simulink model "SWC_FDC_type"  (R2021b)
settings: Solver=FixedStepDiscrete  StartTime=0.0  StopTime=10.0  FixedStep=0.001  RelTol=1e-3
values from neighbouring files (symbols this model uses):
  DID_VCUKey = uint16(0x0202)    [vcu_local_hdr.m]
  DID_XWD = uint16(513)    [vcu_local_hdr.m]
  DIDLen_APSFunConfig = uint16(16)    [vcu_local_hdr.m]
  DIDLen_AutoLock = uint16(1)    [vcu_local_hdr.m]
  DIDLen_DKCKey = uint16(8)    [vcu_local_hdr.m]
  DIDLen_DRLDis = uint16(1)    [vcu_local_hdr.m]
  DIDLen_DynoMode = uint16(1)    [vcu_local_hdr.m]
  DIDLen_FMHTimer = uint16(1)    [vcu_local_hdr.m]
  DIDLen_LFLowPresThre = uint16(1)    [vcu_local_hdr.m]
  DIDLen_LFSensorID = uint16(4)    [vcu_local_hdr.m]
  DIDLen_LRLowPresThre = uint16(1)    [vcu_local_hdr.m]
  DIDLen_LRSensorID = uint16(4)    [vcu_local_hdr.m]
  DIDLen_RFLowPresThre = uint16(1)    [vcu_local_hdr.m]
  DIDLen_RFSensorID = uint16(4)    [vcu_local_hdr.m]
  DIDLen_RRLowPresThre = uint16(1)    [vcu_local_hdr.m]
  DIDLen_RRSensorID = uint16(4)    [vcu_local_hdr.m]
  DIDLen_SensorMode = uint16(1)    [vcu_local_hdr.m]
  DIDLen_TireSize = uint16(16)    [vcu_local_hdr.m]
  DIDLen_TPMSLearnSta = uint16(1)    [vcu_local_hdr.m]
  DIDLen_TurnLampFLThreCurr = uint16(1)    [vcu_local_hdr.m]
  DIDLen_TurnLampFRThreCurr = uint16(1)    [vcu_local_hdr.m]
  DIDLen_TurnLampRLThreCurr = uint16(1)    [vcu_local_hdr.m]
  DIDLen_TurnLampRRThreCurr = uint16(1)    [vcu_local_hdr.m]
  DIDLen_USSConfig = uint16(16)    [vcu_local_hdr.m]
  DIDLen_WhlPres = uint16(4)    [vcu_local_hdr.m]
  DIDLen_WhlSensorBattSta = uint16(1)    [vcu_local_hdr.m]
  DIDLen_WhlTmp = uint16(4)    [vcu_local_hdr.m]
  DIDLen_XWDMode = uint16(1)    [vcu_local_hdr.m]
  DIDNum_APSFunConfig = uint16(0x0903)    [vcu_local_hdr.m]
  DIDNum_AutoLock = uint16(0x0306)    [vcu_local_hdr.m]
  DIDNum_DKCKey = uint16(0x0202)    [vcu_local_hdr.m]
  DIDNum_DRLDis = uint16(0x0307)    [vcu_local_hdr.m]
  DIDNum_DynoMode = uint16(0x0203)    [vcu_local_hdr.m]
  DIDNum_FMHTimer = uint16(0x0305)    [vcu_local_hdr.m]
  DIDNum_LFLowPresThre = uint16(0x0B08)    [vcu_local_hdr.m]
  DIDNum_LFSensorID = uint16(0x0B01)    [vcu_local_hdr.m]
  DIDNum_LRLowPresThre = uint16(0x0B0A)    [vcu_local_hdr.m]
  DIDNum_LRSensorID = uint16(0x0B03)    [vcu_local_hdr.m]
  DIDNum_RFLowPresThre = uint16(0x0B09)    [vcu_local_hdr.m]
  DIDNum_RFSensorID = uint16(0x0B02)    [vcu_local_hdr.m]
  DIDNum_RRLowPresThre = uint16(0x0B0B)    [vcu_local_hdr.m]
  DIDNum_RRSensorID = uint16(0x0B04)    [vcu_local_hdr.m]
  DIDNum_SensorMode = uint16(0x0B0C)    [vcu_local_hdr.m]
  DIDNum_TireSize = uint16(0x0902)    [vcu_local_hdr.m]
  DIDNum_TPMSLearnSta = uint16(0x0B0D)    [vcu_local_hdr.m]
  DIDNum_TurnLampFLThreCurr = uint16(0x0303)    [vcu_local_hdr.m]
  DIDNum_TurnLampFRThreCurr = uint16(0x0301)    [vcu_local_hdr.m]
  DIDNum_TurnLampRLThreCurr = uint16(0x0304)    [vcu_local_hdr.m]
  DIDNum_TurnLampRRThreCurr = uint16(0x0302)    [vcu_local_hdr.m]
  DIDNum_USSConfig = uint16(0x0901)    [vcu_local_hdr.m]
  DIDNum_WhlPres = uint16(0x0B05)    [vcu_local_hdr.m]
  DIDNum_WhlSensorBattSta = uint16(0x0B07)    [vcu_local_hdr.m]
  DIDNum_WhlTmp = uint16(0x0B06)    [vcu_local_hdr.m]
  DIDNum_XWDMode = uint16(0x0201)    [vcu_local_hdr.m]
  DIDVCUKeyLength = uint16(8)    [vcu_local_hdr.m]
  ENUM_DRIVETRAIN_AWD = uint8(  2  )    [vcu_local_hdr.m]
  ENUM_DRIVETRAIN_FWD = uint8(  1  )    [vcu_local_hdr.m]
  ENUM_DRIVETRAIN_RWD = uint8(  0  )    [vcu_local_hdr.m]
  ENUM_REGENLEVEL_INVALID = uint8(  7  )    [vcu_local_hdr.m]
  ENUM_REGENLEVEL_LV1 = uint8(  1  )    [vcu_local_hdr.m]
  ENUM_REGENLEVEL_LV2 = uint8(  2  )    [vcu_local_hdr.m]
  ENUM_REGENLEVEL_LV3 = uint8(  3  )    [vcu_local_hdr.m]
  ENUM_REGENLEVEL_LV4 = uint8(  4  )    [vcu_local_hdr.m]
  ENUM_REGENLEVEL_LV5 = uint8(  5  )    [vcu_local_hdr.m]
  ENUM_REGENLEVEL_OFF = uint8(  0  )    [vcu_local_hdr.m]
  ENUM_REGENLEVEL_OPD = uint8(  6  )    [vcu_local_hdr.m]
  ENUM_TPMSLearnStatus_LEARNED = uint8(  1  )    [vcu_local_hdr.m]
  ENUM_TPMSLearnStatus_LEARNFAIL = uint8(  2  )    [vcu_local_hdr.m]
  ENUM_TPMSLearnStatus_NOTLEARN = uint8(  0  )    [vcu_local_hdr.m]
  ENUM_TPMSSTA_FAT = uint8(  8  )    [vcu_local_hdr.m]
  ENUM_TPMSSTA_LOWBATTERY = uint8(  2  )    [vcu_local_hdr.m]
  FALSE = boolean( 0 )    [vcu_local_hdr.m]
  ONE_INT = uint8(1)    [vcu_local_hdr.m]
  P_boolean = 0.0    [APPTypes.sldd]
  TRUE = boolean( 1 )    [vcu_local_hdr.m]
  ZERO_FLOAT = single(0)    [vcu_local_hdr.m]
  ZERO_INT = uint8(0)    [vcu_local_hdr.m]
undefined symbols (not defined in the file or in its folder): f32_ApsOutVehSpdSig, KHAL_DKCDecryptEnable_flg_ovrdflg, KHAL_DKCDecryptEnable_flg_ovrdval, KHAL_RandomNumberY1_enum, KHAL_RandomNumberY2_enum, KHAL_RandomNumberY_ovrdflg, KHAL_THCMAPTCWarningDTC_flg_ovrdflg, KHAL_THCMAPTCWarningDTC_flg_ovrdval, KHAL_TPMSRESBUTT_flg_ovrdflg, KHAL_TPMSRESBUTT_flg_ovrdval, R_DIDWriteCDD_CSOP_DIDSet_APSFunConfig, R_DIDWriteCDD_CSOP_DIDSet_AutoLock, R_DIDWriteCDD_CSOP_DIDSet_DKCKey, R_DIDWriteCDD_CSOP_DIDSet_DRLDis, R_DIDWriteCDD_CSOP_DIDSet_DynoMode, R_DIDWriteCDD_CSOP_DIDSet_FMHTimer, R_DIDWriteCDD_CSOP_DIDSet_LFLowPresThre, R_DIDWriteCDD_CSOP_DIDSet_LFSensorID, R_DIDWriteCDD_CSOP_DIDSet_LRLowPresThre, R_DIDWriteCDD_CSOP_DIDSet_LRSensorID, R_DIDWriteCDD_CSOP_DIDSet_RFLowPresThre, R_DIDWriteCDD_CSOP_DIDSet_RFSensorID, R_DIDWriteCDD_CSOP_DIDSet_RRLowPresThre, R_DIDWriteCDD_CSOP_DIDSet_RRSensorID, R_DIDWriteCDD_CSOP_DIDSet_SensorMode, R_DIDWriteCDD_CSOP_DIDSet_TireSize, R_DIDWriteCDD_CSOP_DIDSet_TPMSLearnSta, R_DIDWriteCDD_CSOP_DIDSet_TurnLampFLThreCurr, R_DIDWriteCDD_CSOP_DIDSet_TurnLampFRThreCurr, R_DIDWriteCDD_CSOP_DIDSet_TurnLampRLThreCurr, R_DIDWriteCDD_CSOP_DIDSet_TurnLampRRThreCurr, R_DIDWriteCDD_CSOP_DIDSet_USSConfig, R_DIDWriteCDD_CSOP_DIDSet_WhlPres, R_DIDWriteCDD_CSOP_DIDSet_WhlSensorBattSta, R_DIDWriteCDD_CSOP_DIDSet_WhlTmp, R_DIDWriteCDD_CSOP_DIDSet_XWDMode, R_E2E_CAN3_VCU1_CSOP_Write_CAN3_VCU1, R_E2E_CAN3_VCU1_toNIDEC_CSOP_Write_CAN3_VCU1_toNIDEC, R_E2E_CAN4_VCU1_CSOP_Write_CAN4_VCU1, R_FDCCDD_Inner_CSOP_FDC_AppCallSleep, R_HALINCDD_CSOP_PAS_Handler, R_HALINCDD_CSOP_UDS_Main, R_HALOUT_APS_CSOP_ApsOutput, R_HALOUTCDD_CSOP_AppNmStateReq, R_HALOUTCDD_CSOP_SetAcoreRebootCmdACK, R_HALOUTCDD_CSOP_SetSysPwrStat, R_HALOUTCDD_CSOP_SleepRequest, R_IOExpOUT_CDD_CSOP_IOExpSetVal, R_NVMReadCDD_Inner_NVM_ReadOperation, R_NVMWriteCDD_Inner_NVM_WriteOperation, R_UDSCDD_CSOP_DdmRestartOperationCycle, R_WDGCDD_CSOP_Call_Watchdog, R_WDGCDD_CSOP_Call_WDG_AppEnd, R_WDGCDD_CSOP_Call_WDG_AppStart, u16_DIDLen_APSFunConfig, u16_DIDLen_AutoLock, u16_DIDLen_DKCKey, u16_DIDLen_DRLDis, u16_DIDLen_DynoMode, u16_DIDLen_FMHTimer ... (+83)
libraries: simulink x215, FVT_lib x139, hcu_lib x21, hdlsllib x9, app x1, halin x1, halout x1, inp x1, outp x1
(part 8 of 12)

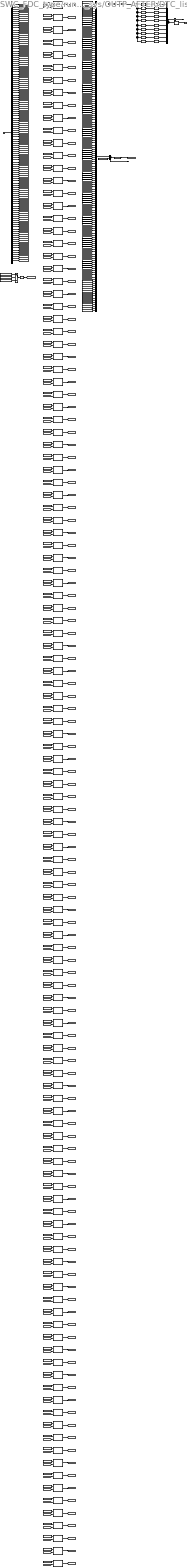
== system SWC_FDC_type/run_SWC_FDC_RxTx_5ms_sys/OUTP_AFTER/DTC_list ==
  BOUTP_outputs : Inport
  BitwiseAND : simulink/Logic and Bit Operations/Bitwise Operator  logicop=AND  UseBitMask=on  BitMask=0x0001  BitMaskRealWorld=Stored Integer
  Constant{,1..22} (23 alike) : Constant  Value=ZERO_INT  OutDataTypeStr=uint32
  Constant23 : Constant  Value=[0 0 0 0 0 0 0 0 0 0 0 0 0 0 0 0 0 0 0 0 0 0 0 0 0 0 0 0 0 0 0 0 0 0 0 0 0 0 0 0 0 0 0 0 0 0 0 0 0 0 0 0 0 0 0 0 0 0 0 0 0 0 0 0 0 0 0 0 0 0 0 0 0 0 0 0 0 0 0 0 0 0 0 0 0 0 0 0 0 0 0 0 0 0 0 0 0 0 0 0 0 0 0 0 0 0 0 0 0 0 0 0 0 0 0 0 0 0 0 0 0 0 0 0 0 0 0 0 0 0 0 0 0 0 0 0 0 0 0 0 0 0 0 0 0 0 0 0 0 0 0 0 0 0 0 0 0 0 0 0 0 0 0 0 0 0 0 0 0 0 0 0]  OutDataTypeStr=uint32
  Constant24 : DataTypeConversion
  Constant25 : Constant  Value=KHAL_THCMAPTCWarningDTC_flg_ovrdflg
  Constant26 : Constant  Value=FALSE
  Constant27 : Constant  Value=KHAL_THCMAPTCWarningDTC_flg_ovrdval
  DTCHeader{,1..9} (10 alike) : FVT_lib/hal/DTC_Header
  DTCID : Constant  Value=0x900909
  DTCID+Status{,1..124} (125 alike) : FVT_lib/hal/DTC_ID_and_Info
  DTCID1 : Constant  Value=0x90090A
  DTCID10 : Constant  Value=0x900913
  DTCID100 : Constant  Value=0x100248
  DTCID101 : Constant  Value=0x100249
  DTCID102 : Constant  Value=0x100250
  DTCID103 : Constant  Value=0x100251
  DTCID104 : Constant  Value=0x100252
  DTCID105 : Constant  Value=0x900253
  DTCID106 : Constant  Value=0x900254
  DTCID107 : Constant  Value=0xD00A01
  DTCID108 : Constant  Value=0xD00A02
  DTCID109 : Constant  Value=0xD00A03
  DTCID11 : Constant  Value=0x900914
  DTCID110 : Constant  Value=0xD00A04
  DTCID111 : Constant  Value=0xD00A05
  DTCID112 : Constant  Value=0xD00A06
  DTCID113 : Constant  Value=0xD00A07
  DTCID114 : Constant  Value=0xD00A0B
  DTCID115 : Constant  Value=0xD00A0C
  DTCID116 : Constant  Value=0xD00A0D
  DTCID117 : Constant  Value=0xD00A0E
  DTCID118 : Constant  Value=0x100A10
  DTCID119 : Constant  Value=0x100A12
  DTCID12 : Constant  Value=0x500B01
  DTCID120 : Constant  Value=0x100A16
  DTCID121 : Constant  Value=0x100A17
  DTCID122 : Constant  Value=0x100A18
  DTCID123 : Constant  Value=0x100A19
  DTCID124 : Constant  Value=0x900401
  DTCID13 : Constant  Value=0x500B02
  DTCID14 : Constant  Value=0x500B03
  DTCID15 : Constant  Value=0x500B04
  DTCID16 : Constant  Value=0x500B05
  DTCID17 : Constant  Value=0x500B06
  DTCID18 : Constant  Value=0x500B07
  DTCID19 : Constant  Value=0x500B08
  DTCID2 : Constant  Value=0x90090B
  DTCID20 : Constant  Value=0x500B09
  DTCID21 : Constant  Value=0x500B0A
  DTCID22 : Constant  Value=0x500B0B
  DTCID23 : Constant  Value=0x500B0C
  DTCID24 : Constant  Value=0x500B0D
  DTCID25 : Constant  Value=0x500B0E
  DTCID26 : Constant  Value=0x500B0F
  DTCID27 : Constant  Value=0x500B10
  DTCID28 : Constant  Value=0x900301
  DTCID29 : Constant  Value=0x900302
  DTCID3 : Constant  Value=0x90090C
  DTCID30 : Constant  Value=0x900303
  DTCID31 : Constant  Value=0x900304
  DTCID32 : Constant  Value=0x900305
  DTCID33 : Constant  Value=0xD00201
  DTCID34 : Constant  Value=0xD00202
  DTCID35 : Constant  Value=0xD00203
  DTCID36 : Constant  Value=0xD00204
  DTCID37 : Constant  Value=0xD00205
  DTCID38 : Constant  Value=0xD00206
  DTCID39 : Constant  Value=0xD00207
  DTCID4 : Constant  Value=0x90090D
  DTCID40 : Constant  Value=0xD00208
  DTCID41 : Constant  Value=0xD00209
  DTCID42 : Constant  Value=0xD0020A
  DTCID43 : Constant  Value=0x10020B
  DTCID44 : Constant  Value=0x10020C
  DTCID45 : Constant  Value=0x10020D
  DTCID46 : Constant  Value=0x10020E
  DTCID47 : Constant  Value=0x100210
  DTCID48 : Constant  Value=0x100211
  DTCID49 : Constant  Value=0x100212
  DTCID5 : Constant  Value=0x90090E
  DTCID50 : Constant  Value=0x100213
  DTCID51 : Constant  Value=0x100214
  DTCID52 : Constant  Value=0x100215
  DTCID53 : Constant  Value=0x100216
  DTCID54 : Constant  Value=0x100217
  DTCID55 : Constant  Value=0x100218
  DTCID56 : Constant  Value=0x100219
  DTCID57 : Constant  Value=0x10021A
  DTCID58 : Constant  Value=0x10021B
  DTCID59 : Constant  Value=0x10021C
  DTCID6 : Constant  Value=0x90090F
  DTCID60 : Constant  Value=0x10021D
  DTCID61 : Constant  Value=0x10021E
  DTCID62 : Constant  Value=0x90021F
  DTCID63 : Constant  Value=0x100220
  DTCID64 : Constant  Value=0x100221
  DTCID65 : Constant  Value=0x100223
  DTCID66 : Constant  Value=0x100224
  DTCID67 : Constant  Value=0x100225
  DTCID68 : Constant  Value=0x100226
  DTCID69 : Constant  Value=0x100227
  DTCID7 : Constant  Value=0x900910
  DTCID70 : Constant  Value=0xD00228
  DTCID71 : Constant  Value=0xD00229
  DTCID72 : Constant  Value=0xD0022A
  DTCID73 : Constant  Value=0xD0022B
  DTCID74 : Constant  Value=0xD0022C
  DTCID75 : Constant  Value=0xD0022D
  DTCID76 : Constant  Value=0x90022E
  DTCID77 : Constant  Value=0x90022F
  DTCID78 : Constant  Value=0xD00230
  DTCID79 : Constant  Value=0xD00231
  DTCID8 : Constant  Value=0x900911
  DTCID80 : Constant  Value=0xD00232
  DTCID81 : Constant  Value=0xD00233
  DTCID82 : Constant  Value=0xD00234
  DTCID83 : Constant  Value=0xD00235
  DTCID84 : Constant  Value=0xD00236
  DTCID85 : Constant  Value=0xD00237
  DTCID86 : Constant  Value=0xD00238
  DTCID87 : Constant  Value=0xD00239
  DTCID88 : Constant  Value=0xD0023A
  DTCID89 : Constant  Value=0xD0023B
  DTCID9 : Constant  Value=0x900912
  DTCID90 : Constant  Value=0xD0023C
  DTCID91 : Constant  Value=0xD0023D
  DTCID92 : Constant  Value=0xD0023E
  DTCID93 : Constant  Value=0xD0023F
  DTCID94 : Constant  Value=0xD00240
  DTCID95 : Constant  Value=0xD00241
  DTCID96 : Constant  Value=0x100242
  DTCID97 : Constant  Value=0x100243
  DTCID98 : Constant  Value=0x100244
  DTCID99 : Constant  Value=0x100247
  Data Type Conversion : DataTypeConversion  OutDataTypeStr=uint32
  Mux : Mux  Inputs=148
  Mux1 : Mux  Inputs=2
  Mux2 : Mux  Inputs=10
  OR : Logic  Operator=OR  Inputs=1  AllPortsSameDT=off  OutDataTypeStr=boolean
  Selector : Selector  InputPortWidth=320  IndexOptions=Index vector (dialog)  Indices=[1:32]  OutputSizes=1
  Selector1 : Selector  InputPortWidth=320  IndexOptions=Index vector (dialog)  Indices=[33:64]  OutputSizes=1
  Selector2 : Selector  InputPortWidth=320  IndexOptions=Index vector (dialog)  Indices=[65:96]  OutputSizes=1
  Selector3 : Selector  InputPortWidth=320  IndexOptions=Index vector (dialog)  Indices=[97:128]  OutputSizes=1
  Selector4 : Selector  InputPortWidth=320  IndexOptions=Index vector (dialog)  Indices=[129:160]  OutputSizes=1
  Selector5 : Selector  InputPortWidth=320  IndexOptions=Index vector (dialog)  Indices=[161:192]  OutputSizes=1
  Selector6 : Selector  InputPortWidth=320  IndexOptions=Index vector (dialog)  Indices=[193:224]  OutputSizes=1
  Selector7 : Selector  InputPortWidth=320  IndexOptions=Index vector (dialog)  Indices=[225:256]  OutputSizes=1
  Selector8 : Selector  InputPortWidth=320  IndexOptions=Index vector (dialog)  Indices=[257:288]  OutputSizes=1
  Selector9 : Selector  InputPortWidth=320  IndexOptions=Index vector (dialog)  Indices=[289:320]  OutputSizes=1
  Switch : Switch  Criteria=u2 > Threshold
  UnitConverter : DataTypeConversion
  bus_selector : BusSelector  OutputSignals=VOUTP_FCLUSSDTC_raw32,VOUTP_FMLUSSDTC_raw32,VOUTP_FMRUSSDTC_raw32,VOUTP_FCRUSSDTC_raw32,VOUTP_RCLUSSDTC_raw32,VOUTP_RMLUSSDTC_raw32,VOUTP_RMRUSSDTC_raw32,VOUTP_RCRUSSDTC_raw32,VOUTP_FLLUSSDTC_raw32,VOUTP_FLRUSSDTC_raw32,VOUTP_RLLUSSDTC_raw32,VOUTP_RLRUSSDTC_raw32,VOUTP_LFPressIndiDTC_raw32,VOUTP_RFPressIndiDTC_raw32,VOUTP_LRPressIndiDTC_raw32,VOUTP_RRPressIndiDTC_raw32,VOUTP_LFWheelTmpHighDTC_raw32,VOUTP_RFWheelTmpHighDTC_raw32,VOUTP_LRWheelTmpHighDTC_raw32,VOUTP_RRWheelTmpHighDTC_raw32,VOUTP_LFBatwarnDTC_raw32,VOUTP_RFBatwarnDTC_raw32,VOUTP_LRBatwarnDTC_raw32,VOUTP_RRBatwarnDTC_raw32,VOUTP_LFSensorFailDTC_raw32,VOUTP_RFSensorFailDTC_raw32,VOUTP_LRSensorFailDTC_raw32,VOUTP_RRSensorFailDTC_raw32,VOUTP_DiagFRTSDTC_raw32,VOUTP_DiagRRTSDTC_raw32,VOUTP_DiagFLTSDTC_raw32,VOUTP_DiagRLTSDTC_raw32,VOUTP_DiagHCrashDTC_raw32,VOUTP_C3BMS6RCDTC_raw32,VOUTP_C3BMS6CSDTC_raw32,VOUTP_C3BMS1RCDTC_raw32,VOUTP_C3BMS1CSDTC_raw32,VOUTP_C3CCU1RCDTC_raw32,VOUTP_C3CCU1CSDTC_raw32,VOUTP_C3CCU2RCDTC_raw32,VOUTP_C3CCU2CSDTC_raw32,VOUTP_C1ABM1RCDTC_raw32,VOUTP_C1ABM1CSDTC_raw32,VOUTP_Lv1ErrDTC_raw32,VOUTP_Lv2ErrDTC_raw32,VOUTP_Lv3ErrDTC_raw32,VOUTP_Lv4ErrDTC_raw32,VOUTP_IniLVLoDTC_raw32,VOUTP_LVSupHiDTC_raw32,VOUTP_LVSupLoDTC_raw32,VOUTP_HVB4PreDTC_raw32,VOUTP_MCU4PreDTC_raw32,VOUTP_DCDC4PreDTC_raw32,VOUTP_HVRlyCloDTC_raw32,VOUTP_BMSRdyDTC_raw32,VOUTP_DCDCEnaDTC_raw32,VOUTP_HiLvSaChkDTC_raw32,VOUTP_MidLvSaChkDTC_raw32,VOUTP_MCUDisDTC_raw32,VOUTP_DCDCDisDTC_raw32,VOUTP_HVRlyOpDTC_raw32,VOUTP_MCUActDTC_raw32,VOUTP_OBC4PreDTC_raw32,VOUTP_BrkSWErrDTC_raw32,VOUTP_BrkSWNoBacDTC_raw32,VOUTP_DrStSWDTC_raw32,VOUTP_FLDoorSWDTC_raw32,VOUTP_FRDoorSWDTC_raw32,VOUTP_RLDoorSWDTC_raw32,VOUTP_RRDoorSWDTC_raw32,VOUTP_C3BMS6LCDTC_raw32,VOUTP_C3BMS1LCDTC_raw32,VOUTP_C3CCU1LCDTC_raw32,VOUTP_C3CCU2LCDTC_raw32,VOUTP_C1ABM1LCDTC_raw32,VOUTP_KeyAuthDTC_raw32,VOUTP_ONtoRdyDTC_raw32,VOUTP_MCUR1NoComDTC_raw32,VOUTP_MCUF1NoComDTC_raw32,VOUTP_Shifter1NoComDTC_raw32,VOUTP_ESC7NoComDTC_raw32,VOUTP_ESC1NoComDTC_raw32,VOUTP_ESC5NoComDTC_raw32,VOUTP_MCUR1RCErrDTC_raw32,VOUTP_MCUF1RCErrDTC_raw32,VOUTP_Shifter1RCErrDTC_raw32,VOUTP_ESC7RCErrDTC_raw32,VOUTP_ESC1RCErrDTC_raw32,VOUTP_ESC5RCErrDTC_raw32,VOUTP_MCUR1CSErrDTC_raw32,VOUTP_MCUF1CSErrDTC_raw32,VOUTP_Shifter1CSErrDTC_raw32,VOUTP_ESC7CSErrDTC_raw32,VOUTP_ESC1CSErrDTC_raw32,VOUTP_ESC5CSErrDTC_raw32,VOUTP_APS1SigOoRDTC_raw32,VOUTP_APS2SigOoRDTC_raw32,VOUTP_APSCorrErrDTC_raw32,VOUTP_5vAPS1PwrErrDTC_raw32,VOUTP_5vAPS2PwrErrDTC_raw32,VOUTP_FrMCUTqErrDTC_raw32,VOUTP_RrMCUTqErrDTC_raw32,VOUTP_EPBLockTODTC_raw32,VOUTP_EPBUnlockTODTC_raw32,VOUTP_HoodSWDTC_raw32,VOUTP_TailgaSWDTC_raw32,VOUTP_FCM2NoComDTC_raw32,VOUTP_FCM3NoComDTC_raw32,VOUTP_FCM4NoComDTC_raw32,VOUTP_FCM5NoComDTC_raw32,VOUTP_ZoneSCPNoComDTC_raw32,VOUTP_FCM2RCErrDTC_raw32,VOUTP_FCM3RCErrDTC_raw32,VOUTP_FCM2CSErrDTC_raw32,VOUTP_FCM3CSErrDTC_raw32,VOUTP_FCM4CSErrDTC_raw32,VOUTP_FCM5CSErrDTC_raw32,VOUTP_BMSSigErrDetDTC_raw32,VOUTP_FCMACCSigErrDetDTC_raw32,VOUTP_FrMCUSigErrDetDTC_raw32,VOUTP_RrMCUSigErrDetDTC_raw32,VOUTP_CCUSigErrDetDTC_raw32,VOUTP_ACCAccelCmdErrDetDTC_raw32
  detect_change : simulink/Logic and Bit Operations/Detect Change  vinit=0  OutDataTypeStr=boolean
  Trigger : Outport
  Header_Array : Outport  Port=2
  DTC_Array : Outport  Port=3
  wires:
  BOUTP_outputs/1 -> bus_selector/1
  bus_selector/1 -> [VOUTP_FCLUSSDTC_raw32]  "<VOUTP_FCLUSSDTC_raw32>"
  bus_selector/2 -> [VOUTP_FMLUSSDTC_raw32]  "<VOUTP_FMLUSSDTC_raw32>"
  bus_selector/3 -> [VOUTP_FMRUSSDTC_raw32]  "<VOUTP_FMRUSSDTC_raw32>"
  bus_selector/4 -> [VOUTP_FCRUSSDTC_raw32]  "<VOUTP_FCRUSSDTC_raw32>"
  bus_selector/5 -> [VOUTP_RCLUSSDTC_raw32]  "<VOUTP_RCLUSSDTC_raw32>"
  bus_selector/6 -> [VOUTP_RMLUSSDTC_raw32]  "<VOUTP_RMLUSSDTC_raw32>"
  bus_selector/7 -> [VOUTP_RMRUSSDTC_raw32]  "<VOUTP_RMRUSSDTC_raw32>"
  bus_selector/8 -> [VOUTP_RCRUSSDTC_raw32]  "<VOUTP_RCRUSSDTC_raw32>"
  bus_selector/9 -> [VOUTP_FLLUSSDTC_raw32]  "<VOUTP_FLLUSSDTC_raw32>"
  bus_selector/10 -> [VOUTP_FLRUSSDTC_raw32]  "<VOUTP_FLRUSSDTC_raw32>"
  bus_selector/11 -> [VOUTP_RLLUSSDTC_raw32]  "<VOUTP_RLLUSSDTC_raw32>"
  bus_selector/12 -> [VOUTP_RLRUSSDTC_raw32]  "<VOUTP_RLRUSSDTC_raw32>"
  bus_selector/13 -> [VOUTP_LFPressIndiDTC_raw32]  "<VOUTP_LFPressIndiDTC_raw32>"
  bus_selector/14 -> [VOUTP_RFPressIndiDTC_raw32]  "<VOUTP_RFPressIndiDTC_raw32>"
  bus_selector/15 -> [VOUTP_LRPressIndiDTC_raw32]  "<VOUTP_LRPressIndiDTC_raw32>"
  bus_selector/16 -> [VOUTP_RRPressIndiDTC_raw32]  "<VOUTP_RRPressIndiDTC_raw32>"
  bus_selector/17 -> [VOUTP_LFWheelTmpHighDTC_raw32]  "<VOUTP_LFWheelTmpHighDTC_raw32>"
  bus_selector/18 -> [VOUTP_RFWheelTmpHighDTC_raw32]  "<VOUTP_RFWheelTmpHighDTC_raw32>"
  bus_selector/19 -> [VOUTP_LRWheelTmpHighDTC_raw32]  "<VOUTP_LRWheelTmpHighDTC_raw32>"
  bus_selector/20 -> [VOUTP_RRWheelTmpHighDTC_raw32]  "<VOUTP_RRWheelTmpHighDTC_raw32>"
  bus_selector/21 -> [VOUTP_LFBatwarnDTC_raw32]  "<VOUTP_LFBatwarnDTC_raw32>"
  bus_selector/22 -> [VOUTP_RFBatwarnDTC_raw32]  "<VOUTP_RFBatwarnDTC_raw32>"
  bus_selector/23 -> [VOUTP_LRBatwarnDTC_raw32]  "<VOUTP_LRBatwarnDTC_raw32>"
  bus_selector/24 -> [VOUTP_RRBatwarnDTC_raw32]  "<VOUTP_RRBatwarnDTC_raw32>"
  bus_selector/25 -> [VOUTP_LFSensorFailDTC_raw32]  "<VOUTP_LFSensorFailDTC_raw32>"
  bus_selector/26 -> [VOUTP_RFSensorFailDTC_raw32]  "<VOUTP_RFSensorFailDTC_raw32>"
  bus_selector/27 -> [VOUTP_LRSensorFailDTC_raw32]  "<VOUTP_LRSensorFailDTC_raw32>"
  bus_selector/28 -> [VOUTP_RRSensorFailDTC_raw32]  "<VOUTP_RRSensorFailDTC_raw32>"
  bus_selector/29 -> [VOUTP_DiagFRTSDTC_raw32]  "<VOUTP_DiagFRTSDTC_raw32>"
  bus_selector/30 -> [VOUTP_DiagRRTSDTC_raw32]  "<VOUTP_DiagRRTSDTC_raw32>"
  bus_selector/31 -> [VOUTP_DiagFLTSDTC_raw32]  "<VOUTP_DiagFLTSDTC_raw32>"
  bus_selector/32 -> [VOUTP_DiagRLTSDTC_raw32]  "<VOUTP_DiagRLTSDTC_raw32>"
  bus_selector/33 -> [VOUTP_DiagHCrashDTC_raw32]  "<VOUTP_DiagHCrashDTC_raw32>"
  bus_selector/34 -> [VOUTP_C3BMS6RCDTC_raw32]  "<VOUTP_C3BMS6RCDTC_raw32>"
  bus_selector/35 -> [VOUTP_C3BMS6CSDTC_raw32]  "<VOUTP_C3BMS6CSDTC_raw32>"
  bus_selector/36 -> [VOUTP_C3BMS1RCDTC_raw32]  "<VOUTP_C3BMS1RCDTC_raw32>"
  bus_selector/37 -> [VOUTP_C3BMS1CSDTC_raw32]  "<VOUTP_C3BMS1CSDTC_raw32>"
  bus_selector/38 -> [VOUTP_C3CCU1RCDTC_raw32]  "<VOUTP_C3CCU1RCDTC_raw32>"
  bus_selector/39 -> [VOUTP_C3CCU1CSDTC_raw32]  "<VOUTP_C3CCU1CSDTC_raw32>"
  bus_selector/40 -> [VOUTP_C3CCU2RCDTC_raw32]  "<VOUTP_C3CCU2RCDTC_raw32>"
  bus_selector/41 -> [VOUTP_C3CCU2CSDTC_raw32]  "<VOUTP_C3CCU2CSDTC_raw32>"
  bus_selector/42 -> [VOUTP_C1ABM1RCDTC_raw32]  "<VOUTP_C1ABM1RCDTC_raw32>"
  bus_selector/43 -> [VOUTP_C1ABM1CSDTC_raw32]  "<VOUTP_C1ABM1CSDTC_raw32>"
  bus_selector/44 -> [VOUTP_Lv1ErrDTC_raw32]  "<VOUTP_Lv1ErrDTC_raw32>"
  bus_selector/45 -> [VOUTP_Lv2ErrDTC_raw32]  "<VOUTP_Lv2ErrDTC_raw32>"
  bus_selector/46 -> [VOUTP_Lv3ErrDTC_raw32]  "<VOUTP_Lv3ErrDTC_raw32>"
  bus_selector/47 -> [VOUTP_Lv4ErrDTC_raw32]  "<VOUTP_Lv4ErrDTC_raw32>"
  bus_selector/48 -> [VOUTP_IniLVLoDTC_raw32]  "<VOUTP_IniLVLoDTC_raw32>"
  bus_selector/49 -> [VOUTP_LVSupHiDTC_raw32]  "<VOUTP_LVSupHiDTC_raw32>"
  bus_selector/50 -> [VOUTP_LVSupLoDTC_raw32]  "<VOUTP_LVSupLoDTC_raw32>"
  bus_selector/51 -> [VOUTP_HVB4PreDTC_raw32]  "<VOUTP_HVB4PreDTC_raw32>"
  bus_selector/52 -> [VOUTP_MCU4PreDTC_raw32]  "<VOUTP_MCU4PreDTC_raw32>"
  bus_selector/53 -> [VOUTP_DCDC4PreDTC_raw32]  "<VOUTP_DCDC4PreDTC_raw32>"
  bus_selector/54 -> [VOUTP_HVRlyCloDTC_raw32]  "<VOUTP_HVRlyCloDTC_raw32>"
  bus_selector/55 -> [VOUTP_BMSRdyDTC_raw32]  "<VOUTP_BMSRdyDTC_raw32>"
  bus_selector/56 -> [VOUTP_DCDCEnaDTC_raw32]  "<VOUTP_DCDCEnaDTC_raw32>"
  bus_selector/57 -> [VOUTP_HiLvSaChkDTC_raw32]  "<VOUTP_HiLvSaChkDTC_raw32>"
  bus_selector/58 -> [VOUTP_MidLvSaChkDTC_raw32]  "<VOUTP_MidLvSaChkDTC_raw32>"
  bus_selector/59 -> [VOUTP_MCUDisDTC_raw32]  "<VOUTP_MCUDisDTC_raw32>"
  bus_selector/60 -> [VOUTP_DCDCDisDTC_raw32]  "<VOUTP_DCDCDisDTC_raw32>"
  bus_selector/61 -> [VOUTP_HVRlyOpDTC_raw32]  "<VOUTP_HVRlyOpDTC_raw32>"
  bus_selector/62 -> [VOUTP_MCUActDTC_raw32]  "<VOUTP_MCUActDTC_raw32>"
  bus_selector/63 -> [VOUTP_OBC4PreDTC_raw32]  "<VOUTP_OBC4PreDTC_raw32>"
  bus_selector/64 -> [VOUTP_BrkSWErrDTC_raw32]  "<VOUTP_BrkSWErrDTC_raw32>"
  bus_selector/65 -> [VOUTP_BrkSWNoBacDTC_raw32]  "<VOUTP_BrkSWNoBacDTC_raw32>"
  bus_selector/66 -> [VOUTP_DrStSWDTC_raw32]  "<VOUTP_DrStSWDTC_raw32>"
  bus_selector/67 -> [VOUTP_FLDoorSWDTC_raw32]  "<VOUTP_FLDoorSWDTC_raw32>"
  bus_selector/68 -> [VOUTP_FRDoorSWDTC_raw32]  "<VOUTP_FRDoorSWDTC_raw32>"
  bus_selector/69 -> [VOUTP_RLDoorSWDTC_raw32]  "<VOUTP_RLDoorSWDTC_raw32>"
  bus_selector/70 -> [VOUTP_RRDoorSWDTC_raw32]  "<VOUTP_RRDoorSWDTC_raw32>"
  bus_selector/71 -> [VOUTP_C3BMS6LCDTC_raw32]  "<VOUTP_C3BMS6LCDTC_raw32>"
  bus_selector/72 -> [VOUTP_C3BMS1LCDTC_raw32]  "<VOUTP_C3BMS1LCDTC_raw32>"
  bus_selector/73 -> [VOUTP_C3CCU1LCDTC_raw32]  "<VOUTP_C3CCU1LCDTC_raw32>"
  bus_selector/74 -> [VOUTP_C3CCU2LCDTC_raw32]  "<VOUTP_C3CCU2LCDTC_raw32>"
  bus_selector/75 -> [VOUTP_C1ABM1LCDTC_raw32]  "<VOUTP_C1ABM1LCDTC_raw32>"
  bus_selector/76 -> [VOUTP_KeyAuthDTC_raw32]  "<VOUTP_KeyAuthDTC_raw32>"
  bus_selector/77 -> [VOUTP_ONtoRdyDTC_raw32]  "<VOUTP_ONtoRdyDTC_raw32>"
  bus_selector/78 -> [VOUTP_MCUR1NoComDTC_raw32]  "<VOUTP_MCUR1NoComDTC_raw32>"
  bus_selector/79 -> [VOUTP_MCUF1NoComDTC_raw32]  "<VOUTP_MCUF1NoComDTC_raw32>"
  bus_selector/80 -> [VOUTP_Shifter1NoComDTC_raw32]  "<VOUTP_Shifter1NoComDTC_raw32>"
  bus_selector/81 -> [VOUTP_ESC7NoComDTC_raw32]  "<VOUTP_ESC7NoComDTC_raw32>"
  bus_selector/82 -> [VOUTP_ESC1NoComDTC_raw32]  "<VOUTP_ESC1NoComDTC_raw32>"
  bus_selector/83 -> [VOUTP_ESC5NoComDTC_raw32]  "<VOUTP_ESC5NoComDTC_raw32>"
  bus_selector/84 -> [VOUTP_MCUR1RCErrDTC_raw32]  "<VOUTP_MCUR1RCErrDTC_raw32>"
  bus_selector/85 -> [VOUTP_MCUF1RCErrDTC_raw32]  "<VOUTP_MCUF1RCErrDTC_raw32>"
  bus_selector/86 -> [VOUTP_Shifter1RCErrDTC_raw32]  "<VOUTP_Shifter1RCErrDTC_raw32>"
  bus_selector/87 -> [VOUTP_ESC7RCErrDTC_raw32]  "<VOUTP_ESC7RCErrDTC_raw32>"
  bus_selector/88 -> [VOUTP_ESC1RCErrDTC_raw32]  "<VOUTP_ESC1RCErrDTC_raw32>"
  bus_selector/89 -> [VOUTP_ESC5RCErrDTC_raw32]  "<VOUTP_ESC5RCErrDTC_raw32>"
  bus_selector/90 -> [VOUTP_MCUR1CSErrDTC_raw32]  "<VOUTP_MCUR1CSErrDTC_raw32>"
  bus_selector/91 -> [VOUTP_MCUF1CSErrDTC_raw32]  "<VOUTP_MCUF1CSErrDTC_raw32>"
  bus_selector/92 -> [VOUTP_Shifter1CSErrDTC_raw32]  "<VOUTP_Shifter1CSErrDTC_raw32>"
  bus_selector/93 -> [VOUTP_ESC7CSErrDTC_raw32]  "<VOUTP_ESC7CSErrDTC_raw32>"
  bus_selector/94 -> [VOUTP_ESC1CSErrDTC_raw32]  "<VOUTP_ESC1CSErrDTC_raw32>"
  bus_selector/95 -> [VOUTP_ESC5CSErrDTC_raw32]  "<VOUTP_ESC5CSErrDTC_raw32>"
  bus_selector/96 -> [VOUTP_APS1SigOoRDTC_raw32]  "<VOUTP_APS1SigOoRDTC_raw32>"
  bus_selector/97 -> [VOUTP_APS2SigOoRDTC_raw32]  "<VOUTP_APS2SigOoRDTC_raw32>"
  bus_selector/98 -> [VOUTP_APSCorrErrDTC_raw32]  "<VOUTP_APSCorrErrDTC_raw32>"
  bus_selector/99 -> [VOUTP_5vAPS1PwrErrDTC_raw32]  "<VOUTP_5vAPS1PwrErrDTC_raw32>"
  bus_selector/100 -> [VOUTP_5vAPS2PwrErrDTC_raw32]  "<VOUTP_5vAPS2PwrErrDTC_raw32>"
  bus_selector/101 -> [VOUTP_FrMCUTqErrDTC_raw32]  "<VOUTP_FrMCUTqErrDTC_raw32>"
  bus_selector/102 -> [VOUTP_RrMCUTqErrDTC_raw32]  "<VOUTP_RrMCUTqErrDTC_raw32>"
  bus_selector/103 -> [VOUTP_EPBLockTODTC_raw32]  "<VOUTP_EPBLockTODTC_raw32>"
  bus_selector/104 -> [VOUTP_EPBUnlockTODTC_raw32]  "<VOUTP_EPBUnlockTODTC_raw32>"
  bus_selector/105 -> [VOUTP_HoodSWDTC_raw32]  "<VOUTP_HoodSWDTC_raw32>"
  bus_selector/106 -> [VOUTP_TailgaSWDTC_raw32]  "<VOUTP_TailgaSWDTC_raw32>"
  bus_selector/107 -> [VOUTP_FCM2NoComDTC_raw32]  "<VOUTP_FCM2NoComDTC_raw32>"
  bus_selector/108 -> [VOUTP_FCM3NoComDTC_raw32]  "<VOUTP_FCM3NoComDTC_raw32>"
  bus_selector/109 -> [VOUTP_FCM4NoComDTC_raw32]  "<VOUTP_FCM4NoComDTC_raw32>"
  bus_selector/110 -> [VOUTP_FCM5NoComDTC_raw32]  "<VOUTP_FCM5NoComDTC_raw32>"
  bus_selector/111 -> [VOUTP_ZoneSCPNoComDTC_raw32]  "<VOUTP_ZoneSCPNoComDTC_raw32>"
  bus_selector/112 -> [VOUTP_FCM2RCErrDTC_raw32]  "<VOUTP_FCM2RCErrDTC_raw32>"
  bus_selector/113 -> [VOUTP_FCM3RCErrDTC_raw32]  "<VOUTP_FCM3RCErrDTC_raw32>"
  bus_selector/114 -> [VOUTP_FCM2CSErrDTC_raw32]  "<VOUTP_FCM2CSErrDTC_raw32>"
  bus_selector/115 -> [VOUTP_FCM3CSErrDTC_raw32]  "<VOUTP_FCM3CSErrDTC_raw32>"
  bus_selector/116 -> [VOUTP_FCM4CSErrDTC_raw32]  "<VOUTP_FCM4CSErrDTC_raw32>"
  bus_selector/117 -> [VOUTP_FCM5CSErrDTC_raw32]  "<VOUTP_FCM5CSErrDTC_raw32>"
  bus_selector/118 -> [VOUTP_BMSSigErrDetDTC_raw32]  "<VOUTP_BMSSigErrDetDTC_raw32>"
  bus_selector/119 -> [VOUTP_FCMACCSigErrDetDTC_raw32]  "<VOUTP_FCMACCSigErrDetDTC_raw32>"
  bus_selector/120 -> [VOUTP_FrMCUSigErrDetDTC_raw32]  "<VOUTP_FrMCUSigErrDetDTC_raw32>"
  bus_selector/121 -> [VOUTP_RrMCUSigErrDetDTC_raw32]  "<VOUTP_RrMCUSigErrDetDTC_raw32>"
  bus_selector/122 -> [VOUTP_CCUSigErrDetDTC_raw32]  "<VOUTP_CCUSigErrDetDTC_raw32>"
  bus_selector/123 -> [VOUTP_ACCAccelCmdErrDetDTC_raw32]  "<VOUTP_ACCAccelCmdErrDetDTC_raw32>"
  DTCID/1 -> DTCID+Status/1
  [VOUTP_FCLUSSDTC_raw32] -> DTCID+Status/2
  DTCID+Status/1 -> [DTC_raw9]
  DTCID1/1 -> DTCID+Status1/1
  [VOUTP_FMLUSSDTC_raw32] -> DTCID+Status1/2
  DTCID+Status1/1 -> [DTC_raw10]
  DTCID2/1 -> DTCID+Status2/1
  [VOUTP_FMRUSSDTC_raw32] -> DTCID+Status2/2
  DTCID+Status2/1 -> [DTC_raw11]
  DTCID3/1 -> DTCID+Status3/1
  [VOUTP_FCRUSSDTC_raw32] -> DTCID+Status3/2
  DTCID+Status3/1 -> [DTC_raw12]
  DTCID4/1 -> DTCID+Status4/1
  [VOUTP_RCLUSSDTC_raw32] -> DTCID+Status4/2
  DTCID+Status4/1 -> [DTC_raw13]
  DTCID5/1 -> DTCID+Status5/1
  [VOUTP_RMLUSSDTC_raw32] -> DTCID+Status5/2
  DTCID+Status5/1 -> [DTC_raw14]
  DTCID6/1 -> DTCID+Status6/1
  [VOUTP_RMRUSSDTC_raw32] -> DTCID+Status6/2
  DTCID+Status6/1 -> [DTC_raw15]
  DTCID7/1 -> DTCID+Status7/1
  [VOUTP_RCRUSSDTC_raw32] -> DTCID+Status7/2
  DTCID+Status7/1 -> [DTC_raw16]
  DTCID8/1 -> DTCID+Status8/1
  [VOUTP_FLLUSSDTC_raw32] -> DTCID+Status8/2
  DTCID+Status8/1 -> [DTC_raw17]
  DTCID9/1 -> DTCID+Status9/1
  [VOUTP_FLRUSSDTC_raw32] -> DTCID+Status9/2
  DTCID+Status9/1 -> [DTC_raw18]
  DTCID10/1 -> DTCID+Status10/1
  [VOUTP_RLLUSSDTC_raw32] -> DTCID+Status10/2
  DTCID+Status10/1 -> [DTC_raw19]
  DTCID11/1 -> DTCID+Status11/1
  [VOUTP_RLRUSSDTC_raw32] -> DTCID+Status11/2
  DTCID+Status11/1 -> [DTC_raw20]
  DTCID12/1 -> DTCID+Status12/1
  [VOUTP_LFPressIndiDTC_raw32] -> DTCID+Status12/2
  DTCID+Status12/1 -> [DTC_raw21]
  DTCID13/1 -> DTCID+Status13/1
  [VOUTP_RFPressIndiDTC_raw32] -> DTCID+Status13/2
  DTCID+Status13/1 -> [DTC_raw22]
  DTCID14/1 -> DTCID+Status14/1
  [VOUTP_LRPressIndiDTC_raw32] -> DTCID+Status14/2
  DTCID+Status14/1 -> [DTC_raw23]
  DTCID15/1 -> DTCID+Status15/1
  [VOUTP_RRPressIndiDTC_raw32] -> DTCID+Status15/2
  DTCID+Status15/1 -> [DTC_raw24]
  DTCID16/1 -> DTCID+Status16/1
  [VOUTP_LFWheelTmpHighDTC_raw32] -> DTCID+Status16/2
  DTCID+Status16/1 -> [DTC_raw25]
  DTCID17/1 -> DTCID+Status17/1
  [VOUTP_RFWheelTmpHighDTC_raw32] -> DTCID+Status17/2
  DTCID+Status17/1 -> [DTC_raw26]
  DTCID18/1 -> DTCID+Status18/1
  [VOUTP_LRWheelTmpHighDTC_raw32] -> DTCID+Status18/2
  DTCID+Status18/1 -> [DTC_raw27]
  DTCID19/1 -> DTCID+Status19/1
  [VOUTP_RRWheelTmpHighDTC_raw32] -> DTCID+Status19/2
  DTCID+Status19/1 -> [DTC_raw28]
  DTCID20/1 -> DTCID+Status20/1
  [VOUTP_LFBatwarnDTC_raw32] -> DTCID+Status20/2
  DTCID+Status20/1 -> [DTC_raw29]
  DTCID21/1 -> DTCID+Status21/1
  [VOUTP_RFBatwarnDTC_raw32] -> DTCID+Status21/2
  DTCID+Status21/1 -> [DTC_raw30]
  DTCID22/1 -> DTCID+Status22/1
  [VOUTP_LRBatwarnDTC_raw32] -> DTCID+Status22/2
  DTCID+Status22/1 -> [DTC_raw31]
  DTCID23/1 -> DTCID+Status23/1
  [VOUTP_RRBatwarnDTC_raw32] -> DTCID+Status23/2
  DTCID+Status23/1 -> [DTC_raw32]
  DTCID24/1 -> DTCID+Status24/1
  [VOUTP_LFSensorFailDTC_raw32] -> DTCID+Status24/2
  DTCID+Status24/1 -> [DTC_raw33]
  DTCID25/1 -> DTCID+Status25/1
  [VOUTP_RFSensorFailDTC_raw32] -> DTCID+Status25/2
  DTCID+Status25/1 -> [DTC_raw34]
  DTCID26/1 -> DTCID+Status26/1
  [VOUTP_LRSensorFailDTC_raw32] -> DTCID+Status26/2
  DTCID+Status26/1 -> [DTC_raw35]
  DTCID27/1 -> DTCID+Status27/1
  [VOUTP_RRSensorFailDTC_raw32] -> DTCID+Status27/2
  DTCID+Status27/1 -> [DTC_raw36]
  DTCID28/1 -> DTCID+Status28/1
  [VOUTP_DiagFRTSDTC_raw32] -> DTCID+Status28/2
  DTCID+Status28/1 -> [DTC_raw37]
  DTCID29/1 -> DTCID+Status29/1
  [VOUTP_DiagRRTSDTC_raw32] -> DTCID+Status29/2
  DTCID+Status29/1 -> [DTC_raw38]
  DTCID30/1 -> DTCID+Status30/1
  [VOUTP_DiagFLTSDTC_raw32] -> DTCID+Status30/2
  DTCID+Status30/1 -> [DTC_raw39]
  DTCID31/1 -> DTCID+Status31/1
  [VOUTP_DiagRLTSDTC_raw32] -> DTCID+Status31/2
  DTCID+Status31/1 -> [DTC_raw40]
  DTCID32/1 -> DTCID+Status32/1
  [VOUTP_DiagHCrashDTC_raw32] -> DTCID+Status32/2
  DTCID+Status32/1 -> [DTC_raw41]
  DTCID33/1 -> DTCID+Status33/1
  [VOUTP_C3BMS6RCDTC_raw32] -> DTCID+Status33/2
  DTCID+Status33/1 -> [DTC_raw42]
  DTCID34/1 -> DTCID+Status34/1
  [VOUTP_C3BMS6CSDTC_raw32] -> DTCID+Status34/2
  DTCID+Status34/1 -> [DTC_raw43]
  DTCID35/1 -> DTCID+Status35/1
  [VOUTP_C3BMS1RCDTC_raw32] -> DTCID+Status35/2
  DTCID+Status35/1 -> [DTC_raw44]
  DTCID36/1 -> DTCID+Status36/1
  [VOUTP_C3BMS1CSDTC_raw32] -> DTCID+Status36/2
  DTCID+Status36/1 -> [DTC_raw45]
  DTCID37/1 -> DTCID+Status37/1
  [VOUTP_C3CCU1RCDTC_raw32] -> DTCID+Status37/2
  DTCID+Status37/1 -> [DTC_raw46]
  DTCID38/1 -> DTCID+Status38/1
  [VOUTP_C3CCU1CSDTC_raw32] -> DTCID+Status38/2
  DTCID+Status38/1 -> [DTC_raw47]
  DTCID39/1 -> DTCID+Status39/1
  [VOUTP_C3CCU2RCDTC_raw32] -> DTCID+Status39/2
  DTCID+Status39/1 -> [DTC_raw48]
  DTCID40/1 -> DTCID+Status40/1
  [VOUTP_C3CCU2CSDTC_raw32] -> DTCID+Status40/2
  DTCID+Status40/1 -> [DTC_raw49]
  DTCID41/1 -> DTCID+Status41/1
  [VOUTP_C1ABM1RCDTC_raw32] -> DTCID+Status41/2
  DTCID+Status41/1 -> [DTC_raw50]
  DTCID42/1 -> DTCID+Status42/1
  [VOUTP_C1ABM1CSDTC_raw32] -> DTCID+Status42/2
  DTCID+Status42/1 -> [DTC_raw51]
  DTCID43/1 -> DTCID+Status43/1
  [VOUTP_Lv1ErrDTC_raw32] -> DTCID+Status43/2
  DTCID+Status43/1 -> [DTC_raw52]
  DTCID44/1 -> DTCID+Status44/1
  [VOUTP_Lv2ErrDTC_raw32] -> DTCID+Status44/2
  DTCID+Status44/1 -> [DTC_raw53]
  DTCID45/1 -> DTCID+Status45/1
  [VOUTP_Lv3ErrDTC_raw32] -> DTCID+Status45/2
  DTCID+Status45/1 -> [DTC_raw54]
  DTCID46/1 -> DTCID+Status46/1
  [VOUTP_Lv4ErrDTC_raw32] -> DTCID+Status46/2
  DTCID+Status46/1 -> [DTC_raw55]
  DTCID47/1 -> DTCID+Status47/1
  [VOUTP_IniLVLoDTC_raw32] -> DTCID+Status47/2
  DTCID+Status47/1 -> [DTC_raw56]
  DTCID48/1 -> DTCID+Status48/1
  [VOUTP_LVSupHiDTC_raw32] -> DTCID+Status48/2
  DTCID+Status48/1 -> [DTC_raw57]
  DTCID49/1 -> DTCID+Status49/1
  [VOUTP_LVSupLoDTC_raw32] -> DTCID+Status49/2
  DTCID+Status49/1 -> [DTC_raw58]
  DTCID50/1 -> DTCID+Status50/1
  [VOUTP_HVB4PreDTC_raw32] -> DTCID+Status50/2
  DTCID+Status50/1 -> [DTC_raw59]
  DTCID51/1 -> DTCID+Status51/1
  [VOUTP_MCU4PreDTC_raw32] -> DTCID+Status51/2
  DTCID+Status51/1 -> [DTC_raw60]
  DTCID52/1 -> DTCID+Status52/1
  [VOUTP_DCDC4PreDTC_raw32] -> DTCID+Status52/2
  DTCID+Status52/1 -> [DTC_raw61]
  DTCID53/1 -> DTCID+Status53/1
  [VOUTP_HVRlyCloDTC_raw32] -> DTCID+Status53/2
  DTCID+Status53/1 -> [DTC_raw62]
  DTCID54/1 -> DTCID+Status54/1
  [VOUTP_BMSRdyDTC_raw32] -> DTCID+Status54/2
  DTCID+Status54/1 -> [DTC_raw63]
  DTCID55/1 -> DTCID+Status55/1
  [VOUTP_DCDCEnaDTC_raw32] -> DTCID+Status55/2
  DTCID+Status55/1 -> [DTC_raw64]
  DTCID56/1 -> DTCID+Status56/1
  [VOUTP_HiLvSaChkDTC_raw32] -> DTCID+Status56/2
  DTCID+Status56/1 -> [DTC_raw65]
  DTCID57/1 -> DTCID+Status57/1
  [VOUTP_MidLvSaChkDTC_raw32] -> DTCID+Status57/2
  DTCID+Status57/1 -> [DTC_raw66]
  DTCID58/1 -> DTCID+Status58/1
  [VOUTP_MCUDisDTC_raw32] -> DTCID+Status58/2
  DTCID+Status58/1 -> [DTC_raw67]
  DTCID59/1 -> DTCID+Status59/1
  [VOUTP_DCDCDisDTC_raw32] -> DTCID+Status59/2
  DTCID+Status59/1 -> [DTC_raw68]
  DTCID60/1 -> DTCID+Status60/1
  [VOUTP_HVRlyOpDTC_raw32] -> DTCID+Status60/2
  DTCID+Status60/1 -> [DTC_raw69]
  DTCID61/1 -> DTCID+Status61/1
  [VOUTP_MCUActDTC_raw32] -> DTCID+Status61/2
  DTCID+Status61/1 -> [DTC_raw70]
  DTCID62/1 -> DTCID+Status62/1
  [VOUTP_OBC4PreDTC_raw32] -> DTCID+Status62/2
  DTCID+Status62/1 -> [DTC_raw71]
  DTCID63/1 -> DTCID+Status63/1
  [VOUTP_BrkSWErrDTC_raw32] -> DTCID+Status63/2
  DTCID+Status63/1 -> [DTC_raw72]
  DTCID64/1 -> DTCID+Status64/1
  [VOUTP_BrkSWNoBacDTC_raw32] -> DTCID+Status64/2
  DTCID+Status64/1 -> [DTC_raw73]
  DTCID65/1 -> DTCID+Status65/1
  [VOUTP_DrStSWDTC_raw32] -> DTCID+Status65/2
  DTCID+Status65/1 -> [DTC_raw74]
  DTCID66/1 -> DTCID+Status66/1
  [VOUTP_FLDoorSWDTC_raw32] -> DTCID+Status66/2
  DTCID+Status66/1 -> [DTC_raw75]
  DTCID67/1 -> DTCID+Status67/1
  [VOUTP_FRDoorSWDTC_raw32] -> DTCID+Status67/2
  DTCID+Status67/1 -> [DTC_raw76]
  DTCID68/1 -> DTCID+Status68/1
  [VOUTP_RLDoorSWDTC_raw32] -> DTCID+Status68/2
  DTCID+Status68/1 -> [DTC_raw77]
  DTCID69/1 -> DTCID+Status69/1
  [VOUTP_RRDoorSWDTC_raw32] -> DTCID+Status69/2
  DTCID+Status69/1 -> [DTC_raw78]
  DTCID70/1 -> DTCID+Status70/1
  [VOUTP_C3BMS6LCDTC_raw32] -> DTCID+Status70/2
  DTCID+Status70/1 -> [DTC_raw79]
  DTCID71/1 -> DTCID+Status71/1
  [VOUTP_C3BMS1LCDTC_raw32] -> DTCID+Status71/2
  DTCID+Status71/1 -> [DTC_raw80]
  DTCID72/1 -> DTCID+Status72/1
  [VOUTP_C3CCU1LCDTC_raw32] -> DTCID+Status72/2
  DTCID+Status72/1 -> [DTC_raw81]
  DTCID73/1 -> DTCID+Status73/1
  [VOUTP_C3CCU2LCDTC_raw32] -> DTCID+Status73/2
  DTCID+Status73/1 -> [DTC_raw82]
  DTCID74/1 -> DTCID+Status74/1
  [VOUTP_C1ABM1LCDTC_raw32] -> DTCID+Status74/2
  DTCID+Status74/1 -> [DTC_raw83]
  DTCID75/1 -> DTCID+Status75/1
  [VOUTP_KeyAuthDTC_raw32] -> DTCID+Status75/2
  DTCID+Status75/1 -> [DTC_raw84]
  DTCID76/1 -> DTCID+Status76/1
  [VOUTP_LVChFrqDTC_raw32] -> DTCID+Status76/2
  DTCID+Status76/1 -> [DTC_raw85]
  DTCID77/1 -> DTCID+Status77/1
  [VOUTP_ONtoRdyDTC_raw32] -> DTCID+Status77/2
  DTCID+Status77/1 -> [DTC_raw86]
  DTCID78/1 -> DTCID+Status78/1
  [VOUTP_MCUR1NoComDTC_raw32] -> DTCID+Status78/2
  DTCID+Status78/1 -> [DTC_raw87]
  DTCID79/1 -> DTCID+Status79/1
  [VOUTP_MCUF1NoComDTC_raw32] -> DTCID+Status79/2
  DTCID+Status79/1 -> [DTC_raw88]
  DTCID80/1 -> DTCID+Status80/1
  [VOUTP_Shifter1NoComDTC_raw32] -> DTCID+Status80/2
  DTCID+Status80/1 -> [DTC_raw89]
  DTCID81/1 -> DTCID+Status81/1
  [VOUTP_ESC7NoComDTC_raw32] -> DTCID+Status81/2
  DTCID+Status81/1 -> [DTC_raw90]
  DTCID82/1 -> DTCID+Status82/1
  [VOUTP_ESC1NoComDTC_raw32] -> DTCID+Status82/2
  DTCID+Status82/1 -> [DTC_raw91]
  DTCID83/1 -> DTCID+Status83/1
  [VOUTP_ESC5NoComDTC_raw32] -> DTCID+Status83/2
  DTCID+Status83/1 -> [DTC_raw92]
  DTCID84/1 -> DTCID+Status84/1
  [VOUTP_MCUR1RCErrDTC_raw32] -> DTCID+Status84/2
  DTCID+Status84/1 -> [DTC_raw93]
  DTCID85/1 -> DTCID+Status85/1
  [VOUTP_MCUF1RCErrDTC_raw32] -> DTCID+Status85/2
  DTCID+Status85/1 -> [DTC_raw94]
  DTCID86/1 -> DTCID+Status86/1
  [VOUTP_Shifter1RCErrDTC_raw32] -> DTCID+Status86/2
  DTCID+Status86/1 -> [DTC_raw95]
  DTCID87/1 -> DTCID+Status87/1
  [VOUTP_ESC7RCErrDTC_raw32] -> DTCID+Status87/2
  DTCID+Status87/1 -> [DTC_raw96]
  DTCID88/1 -> DTCID+Status88/1
  [VOUTP_ESC1RCErrDTC_raw32] -> DTCID+Status88/2
  DTCID+Status88/1 -> [DTC_raw97]
  DTCID89/1 -> DTCID+Status89/1
  [VOUTP_ESC5RCErrDTC_raw32] -> DTCID+Status89/2
  DTCID+Status89/1 -> [DTC_raw98]
  DTCID90/1 -> DTCID+Status90/1
  [VOUTP_MCUR1CSErrDTC_raw32] -> DTCID+Status90/2
  DTCID+Status90/1 -> [DTC_raw99]
  DTCID91/1 -> DTCID+Status91/1
  [VOUTP_MCUF1CSErrDTC_raw32] -> DTCID+Status91/2
  DTCID+Status91/1 -> [DTC_raw100]
  DTCID92/1 -> DTCID+Status92/1
  [VOUTP_Shifter1CSErrDTC_raw32] -> DTCID+Status92/2
  DTCID+Status92/1 -> [DTC_raw101]
  DTCID93/1 -> DTCID+Status93/1
  [VOUTP_ESC7CSErrDTC_raw32] -> DTCID+Status93/2
  DTCID+Status93/1 -> [DTC_raw102]
  DTCID94/1 -> DTCID+Status94/1
  [VOUTP_ESC1CSErrDTC_raw32] -> DTCID+Status94/2
  DTCID+Status94/1 -> [DTC_raw103]
  DTCID95/1 -> DTCID+Status95/1
  [VOUTP_ESC5CSErrDTC_raw32] -> DTCID+Status95/2
  DTCID+Status95/1 -> [DTC_raw104]
  DTCID96/1 -> DTCID+Status96/1
  [VOUTP_APS1SigOoRDTC_raw32] -> DTCID+Status96/2
  DTCID+Status96/1 -> [DTC_raw105]
  DTCID97/1 -> DTCID+Status97/1
  [VOUTP_APS2SigOoRDTC_raw32] -> DTCID+Status97/2
  DTCID+Status97/1 -> [DTC_raw106]
  DTCID98/1 -> DTCID+Status98/1
  [VOUTP_APSCorrErrDTC_raw32] -> DTCID+Status98/2
  DTCID+Status98/1 -> [DTC_raw107]
  DTCID99/1 -> DTCID+Status99/1
  [VOUTP_5vAPS1PwrErrDTC_raw32] -> DTCID+Status99/2
  DTCID+Status99/1 -> [DTC_raw108]
  DTCID100/1 -> DTCID+Status100/1
  [VOUTP_5vAPS2PwrErrDTC_raw32] -> DTCID+Status100/2
  DTCID+Status100/1 -> [DTC_raw109]
  DTCID101/1 -> DTCID+Status101/1
  [VOUTP_FrMCUTqErrDTC_raw32] -> DTCID+Status101/2
  DTCID+Status101/1 -> [DTC_raw110]
  DTCID102/1 -> DTCID+Status102/1
  [VOUTP_RrMCUTqErrDTC_raw32] -> DTCID+Status102/2
  DTCID+Status102/1 -> [DTC_raw111]
  DTCID103/1 -> DTCID+Status103/1
  [VOUTP_EPBLockTODTC_raw32] -> DTCID+Status103/2
  DTCID+Status103/1 -> [DTC_raw112]
  DTCID104/1 -> DTCID+Status104/1
  [VOUTP_EPBUnlockTODTC_raw32] -> DTCID+Status104/2
  DTCID+Status104/1 -> [DTC_raw113]
  DTCID105/1 -> DTCID+Status105/1
  [VOUTP_HoodSWDTC_raw32] -> DTCID+Status105/2
  DTCID+Status105/1 -> [DTC_raw114]
  DTCID106/1 -> DTCID+Status106/1
  [VOUTP_TailgaSWDTC_raw32] -> DTCID+Status106/2
  DTCID+Status106/1 -> [DTC_raw115]
  DTCID107/1 -> DTCID+Status107/1
  [VOUTP_FCM2NoComDTC_raw32] -> DTCID+Status107/2
  DTCID+Status107/1 -> [DTC_raw116]
  DTCID108/1 -> DTCID+Status108/1
  [VOUTP_FCM3NoComDTC_raw32] -> DTCID+Status108/2
  DTCID+Status108/1 -> [DTC_raw117]
  DTCID109/1 -> DTCID+Status109/1
  [VOUTP_FCM4NoComDTC_raw32] -> DTCID+Status109/2
  DTCID+Status109/1 -> [DTC_raw118]
  DTCID110/1 -> DTCID+Status110/1
  [VOUTP_FCM5NoComDTC_raw32] -> DTCID+Status110/2
  DTCID+Status110/1 -> [DTC_raw119]
  DTCID111/1 -> DTCID+Status111/1
  [VOUTP_ZoneSCPNoComDTC_raw32] -> DTCID+Status111/2
  DTCID+Status111/1 -> [DTC_raw120]
  DTCID112/1 -> DTCID+Status112/1
  [VOUTP_FCM2RCErrDTC_raw32] -> DTCID+Status112/2
  DTCID+Status112/1 -> [DTC_raw121]
  DTCID113/1 -> DTCID+Status113/1
  [VOUTP_FCM3RCErrDTC_raw32] -> DTCID+Status113/2
  DTCID+Status113/1 -> [DTC_raw122]
  DTCID114/1 -> DTCID+Status114/1
  [VOUTP_FCM2CSErrDTC_raw32] -> DTCID+Status114/2
  DTCID+Status114/1 -> [DTC_raw123]
  DTCID115/1 -> DTCID+Status115/1
  [VOUTP_FCM3CSErrDTC_raw32] -> DTCID+Status115/2
  DTCID+Status115/1 -> [DTC_raw124]
  DTCID116/1 -> DTCID+Status116/1
  [VOUTP_FCM4CSErrDTC_raw32] -> DTCID+Status116/2
  DTCID+Status116/1 -> [DTC_raw125]
  DTCID117/1 -> DTCID+Status117/1
  [VOUTP_FCM5CSErrDTC_raw32] -> DTCID+Status117/2
  DTCID+Status117/1 -> [DTC_raw126]
  DTCID118/1 -> DTCID+Status118/1
  [VOUTP_BMSSigErrDetDTC_raw32] -> DTCID+Status118/2
  DTCID+Status118/1 -> [DTC_raw127]
  DTCID119/1 -> DTCID+Status119/1
  [VOUTP_FCMACCSigErrDetDTC_raw32] -> DTCID+Status119/2
  DTCID+Status119/1 -> [DTC_raw128]
  DTCID120/1 -> DTCID+Status120/1
  [VOUTP_FrMCUSigErrDetDTC_raw32] -> DTCID+Status120/2
  DTCID+Status120/1 -> [DTC_raw129]
  DTCID121/1 -> DTCID+Status121/1
  [VOUTP_RrMCUSigErrDetDTC_raw32] -> DTCID+Status121/2
  DTCID+Status121/1 -> [DTC_raw130]
  DTCID122/1 -> DTCID+Status122/1
  [VOUTP_CCUSigErrDetDTC_raw32] -> DTCID+Status122/2
  DTCID+Status122/1 -> [DTC_raw131]
  DTCID123/1 -> DTCID+Status123/1
  [VOUTP_ACCAccelCmdErrDetDTC_raw32] -> DTCID+Status123/2
  DTCID+Status123/1 -> [DTC_raw132]
  DTCID124/1 -> DTCID+Status124/1
  [VOUTP_THCMAPTCWarningDTC_raw32] -> DTCID+Status124/2
  DTCID+Status124/1 -> [DTC_raw146]
  Constant/1 -> Mux/1
  Constant1/1 -> Mux/2
  Constant2/1 -> Mux/3
  Constant3/1 -> Mux/4
  Constant4/1 -> Mux/5
  Constant5/1 -> Mux/6
  Constant6/1 -> Mux/7
  Constant7/1 -> Mux/8
  Constant8/1 -> Mux/9
  [DTC_raw9] -> Mux/10
  [DTC_raw10] -> Mux/11
  [DTC_raw11] -> Mux/12
  [DTC_raw12] -> Mux/13
  [DTC_raw13] -> Mux/14
  [DTC_raw14] -> Mux/15
  [DTC_raw15] -> Mux/16
  [DTC_raw16] -> Mux/17
  [DTC_raw17] -> Mux/18
  [DTC_raw18] -> Mux/19
  [DTC_raw19] -> Mux/20
  [DTC_raw20] -> Mux/21
  [DTC_raw21] -> Mux/22
  [DTC_raw22] -> Mux/23
  [DTC_raw23] -> Mux/24
  [DTC_raw24] -> Mux/25
  [DTC_raw25] -> Mux/26
  [DTC_raw26] -> Mux/27
  [DTC_raw27] -> Mux/28
  [DTC_raw28] -> Mux/29
  [DTC_raw29] -> Mux/30
  [DTC_raw30] -> Mux/31
  [DTC_raw31] -> Mux/32
  [DTC_raw32] -> Mux/33
  [DTC_raw33] -> Mux/34
  [DTC_raw34] -> Mux/35
  [DTC_raw35] -> Mux/36
  [DTC_raw36] -> Mux/37
  [DTC_raw37] -> Mux/38
  [DTC_raw38] -> Mux/39
  [DTC_raw39] -> Mux/40
  [DTC_raw40] -> Mux/41
  [DTC_raw41] -> Mux/42
  [DTC_raw42] -> Mux/43
  [DTC_raw43] -> Mux/44
  [DTC_raw44] -> Mux/45
  [DTC_raw45] -> Mux/46
  [DTC_raw46] -> Mux/47
  [DTC_raw47] -> Mux/48
  [DTC_raw48] -> Mux/49
  [DTC_raw49] -> Mux/50
  [DTC_raw50] -> Mux/51
  [DTC_raw51] -> Mux/52
  [DTC_raw52] -> Mux/53
  [DTC_raw53] -> Mux/54
  [DTC_raw54] -> Mux/55
  [DTC_raw55] -> Mux/56
  [DTC_raw56] -> Mux/57
  [DTC_raw57] -> Mux/58
  [DTC_raw58] -> Mux/59
  [DTC_raw59] -> Mux/60
  [DTC_raw60] -> Mux/61
  [DTC_raw61] -> Mux/62
  [DTC_raw62] -> Mux/63
  [DTC_raw63] -> Mux/64
  [DTC_raw64] -> Mux/65
  [DTC_raw65] -> Mux/66
  [DTC_raw66] -> Mux/67
  [DTC_raw67] -> Mux/68
  [DTC_raw68] -> Mux/69
  [DTC_raw69] -> Mux/70
  [DTC_raw70] -> Mux/71
  [DTC_raw71] -> Mux/72
  [DTC_raw72] -> Mux/73
  [DTC_raw73] -> Mux/74
  [DTC_raw74] -> Mux/75
  [DTC_raw75] -> Mux/76
  [DTC_raw76] -> Mux/77
  [DTC_raw77] -> Mux/78
  [DTC_raw78] -> Mux/79
  [DTC_raw79] -> Mux/80
  [DTC_raw80] -> Mux/81
  [DTC_raw81] -> Mux/82
  [DTC_raw82] -> Mux/83
  [DTC_raw83] -> Mux/84
  [DTC_raw84] -> Mux/85
  [DTC_raw85] -> Mux/86
  [DTC_raw86] -> Mux/87
  [DTC_raw87] -> Mux/88
  [DTC_raw88] -> Mux/89
  [DTC_raw89] -> Mux/90
  [DTC_raw90] -> Mux/91
  [DTC_raw91] -> Mux/92
  [DTC_raw92] -> Mux/93
  [DTC_raw93] -> Mux/94
  [DTC_raw94] -> Mux/95
  [DTC_raw95] -> Mux/96
  [DTC_raw96] -> Mux/97
  [DTC_raw97] -> Mux/98
  [DTC_raw98] -> Mux/99
  [DTC_raw99] -> Mux/100
  [DTC_raw100] -> Mux/101
  [DTC_raw101] -> Mux/102
  [DTC_raw102] -> Mux/103
  [DTC_raw103] -> Mux/104
  [DTC_raw104] -> Mux/105
  [DTC_raw105] -> Mux/106
  [DTC_raw106] -> Mux/107
  [DTC_raw107] -> Mux/108
  [DTC_raw108] -> Mux/109
  [DTC_raw109] -> Mux/110
  [DTC_raw110] -> Mux/111
  [DTC_raw111] -> Mux/112
  [DTC_raw112] -> Mux/113
  [DTC_raw113] -> Mux/114
  [DTC_raw114] -> Mux/115
  [DTC_raw115] -> Mux/116
  [DTC_raw116] -> Mux/117
  [DTC_raw117] -> Mux/118
  [DTC_raw118] -> Mux/119
  [DTC_raw119] -> Mux/120
  [DTC_raw120] -> Mux/121
  [DTC_raw121] -> Mux/122
  [DTC_raw122] -> Mux/123
  [DTC_raw123] -> Mux/124
  [DTC_raw124] -> Mux/125
  [DTC_raw125] -> Mux/126
  [DTC_raw126] -> Mux/127
  [DTC_raw127] -> Mux/128
  [DTC_raw128] -> Mux/129
  [DTC_raw129] -> Mux/130
  [DTC_raw130] -> Mux/131
  [DTC_raw131] -> Mux/132
  [DTC_raw132] -> Mux/133
  Constant9/1 -> Mux/134
  Constant10/1 -> Mux/135
  Constant11/1 -> Mux/136
  Constant12/1 -> Mux/137
  Constant13/1 -> Mux/138
  Constant14/1 -> Mux/139
  Constant15/1 -> Mux/140
  Constant16/1 -> Mux/141
  Constant17/1 -> Mux/142
  Constant18/1 -> Mux/143
  Constant19/1 -> Mux/144
  Constant20/1 -> Mux/145
  Constant21/1 -> Mux/146
  [DTC_raw146] -> Mux/147
  Constant22/1 -> Mux/148
  Mux/1 -> Mux1/1
  Constant23/1 -> Mux1/2
  Mux1/1 -> Constant24/1, DTC_Array/1
  Constant24/1 -> [DTC_Array]  "VDTC_DTCArray_raw32"
  [DTC_Array] -> BitwiseAND/1
  BitwiseAND/1 -> detect_change/1
  detect_change/1 -> Selector8/1, Selector9/1, Selector7/1, Selector6/1, Selector5/1, Selector4/1, Selector3/1, Selector2/1, Selector1/1, Selector/1
  Selector/1 -> DTCHeader/1
  DTCHeader/1 -> Mux2/1
  Selector1/1 -> DTCHeader1/1
  DTCHeader1/1 -> Mux2/2
  Selector2/1 -> DTCHeader2/1
  DTCHeader2/1 -> Mux2/3
  Selector3/1 -> DTCHeader3/1
  DTCHeader3/1 -> Mux2/4
  Selector4/1 -> DTCHeader4/1
  DTCHeader4/1 -> Mux2/5
  Selector5/1 -> DTCHeader5/1
  DTCHeader5/1 -> Mux2/6
  Selector6/1 -> DTCHeader6/1
  DTCHeader6/1 -> Mux2/7
  Selector7/1 -> DTCHeader7/1
  DTCHeader7/1 -> Mux2/8
  Selector8/1 -> DTCHeader8/1
  DTCHeader8/1 -> Mux2/9
  Selector9/1 -> DTCHeader9/1
  DTCHeader9/1 -> Mux2/10
  Mux2/1 -> UnitConverter/1, OR/1
  UnitConverter/1 -> Header_Array/1  "VDTC_HeaderArray_raw32"
  OR/1 -> Trigger/1  "VHAL_TriggerDTC_flg"
  Switch/1 -> Data Type Conversion/1
  Constant26/1 -> Switch/3
  Constant25/1 -> Switch/2
  Constant27/1 -> Switch/1
  Data Type Conversion/1 -> [VOUTP_THCMAPTCWarningDTC_raw32]
